simulink model "model"  (R2019a)
settings: Solver=ode15s  StartTime=0.0  StopTime=200  FixedStep=h  MaxStep=0.01  RelTol=1e-3
values from neighbouring files (symbols this model uses):
  d_cart = 4.3726    [parameters.m]
  d_pend = 0.0097    [parameters.m]
  g = 9.81    [parameters.m]
  h = 0.01    [parameters.m]
  Km = 3.7228    [parameters.m]
  l = 0.6    [parameters.m]
  mc = 0.5477    [parameters.m]
  mp = 0.0760    (= 0.076)    [parameters.m]
  sys = ss(A,B,C,D)    [linmod.m]
  ub_mtr_threshold = 0    [parameters.m]
  x_init = [0,0,0,0]    [parameters.m]
undefined symbols (not defined in the file or in its folder): K
libraries: cstblocks x3, mpclib x1
settings Model: Creator=mdepo  LastModifiedBy=mdepo

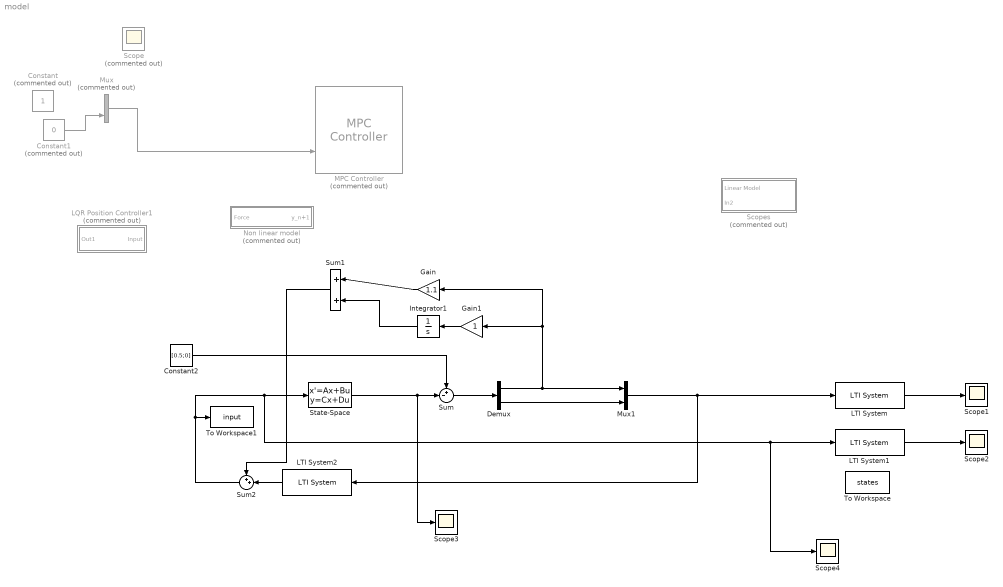
== system model ==
  Constant : Constant  Commented=on
  Constant1 : Constant  Commented=on  Value=0
  Constant2 : Constant  Value=[0.5;0]
  Demux : Demux  Outputs=2
  Gain : Gain  Gain=1.1
  Gain1 : Gain
  Integrator1 : Integrator
  LQR Position Controller1 : Subsystem  Commented=on
  LTI System : cstblocks/LTI System  sys=Ws  IC=[]
  LTI System1 : cstblocks/LTI System  sys=Wu  IC=[]
  LTI System2 : cstblocks/LTI System  sys=K  IC=[]
  MPC Controller : mpclib/MPC Controller  Commented=on  SCDEnableBlockLinearizationSpecification=on  mpcobj=mpcobj  is_multiple=0  enable_value=0  return_u0=off  updateMPCinCallerWorkspace=on  md_inport=off  mv_inport=off  uref_inport=off  return_cost=off  return_mvseq=off  return_qpstatus=off  return_xseq=off  return_state=off  return_ovseq=off  state_inport=off  umin_inport=off  umax_inport=off  ymin_inport=off  ymax_inport=off  cc_inport=off  ywt_inport=off  uwt_inport=off  duwt_inport=off  rhoeps_inport=off  pm_inport=off  MaximumP=10  HorizonChoice=FixedHorizon  n_ts=0.01  n_p=50  n_mv=1  n_md=0  n_ud=0  n_mo=1  n_uo=0  BlockDataType=double  SampleTimeInherited=off  switch_inport=off
      settings: SourceProductName=MATLAB Runtime - Model Predictive Control Toolbox Addin  SourceProductBaseCode=Missing
  Mux : Mux  Commented=on  Inputs=2
  Mux1 : Mux  Inputs=2
  Non linear model : Subsystem  Commented=on
  Scope : Scope  Commented=on
  Scope{1..4} (4 alike) : Scope
  "Scopes " : Subsystem  Commented=on
  State-Space : StateSpace  A=sys.A  B=sys.B  C=sys.C  D=sys.D  InitialCondition=x_init
  Sum : Sum  Inputs=+-|
  Sum1 : Sum  Inputs=|++
  Sum2 : Sum  Inputs=++|
  To Workspace : ToWorkspace  VariableName=states  SampleTime=h
  To Workspace1 : ToWorkspace  VariableName=input  SaveFormat=Timeseries  SampleTime=-1
  wires:
  Constant1/1 -> Mux/2
  Mux/1 -> MPC Controller/2
  LTI System/1 -> Scope1/1
  Constant2/1 -> Sum/1
  State-Space/1 -> Scope3/1, Sum/2
  LTI System1/1 -> Scope2/1
  Sum2/1 -> State-Space/1, Scope4/1, LTI System1/1, To Workspace1/1
  Sum/1 -> Demux/1
  Demux/2 -> Mux1/2
  Mux1/1 -> LTI System2/1, LTI System/1
  Demux/1 -> Gain/1, Gain1/1, Mux1/1
  Gain1/1 -> Integrator1/1
  LTI System2/1 -> Sum2/2
  Sum1/1 -> Sum2/1
  Integrator1/1 -> Sum1/2
  Gain/1 -> Sum1/1

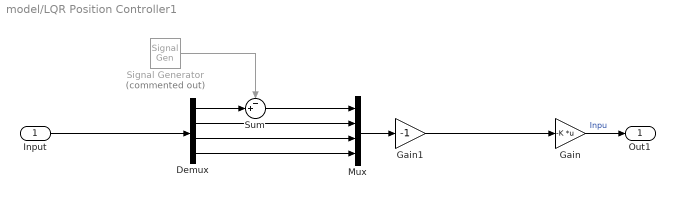
== system model/LQR Position Controller1 ==
  Input : Inport
  Demux : Demux
  Gain : Gain  Gain=-K  Multiplication=Matrix(K*u)
  Gain1 : Gain  Gain=-1
  Mux : Mux
  Signal Generator : SignalGenerator  Commented=on  Units=rad/sec
  Sum : Sum  Inputs=-+|
  Out1 : Outport
  wires:
  Signal Generator/1 -> Sum/1
  Sum/1 -> Mux/1
  Demux/1 -> Sum/2
  Mux/1 -> Gain1/1
  Input/1 -> Demux/1
  Demux/4 -> Mux/4
  Demux/3 -> Mux/3
  Demux/2 -> Mux/2
  Gain/1 -> Out1/1  "Inpu"
  Gain1/1 -> Gain/1

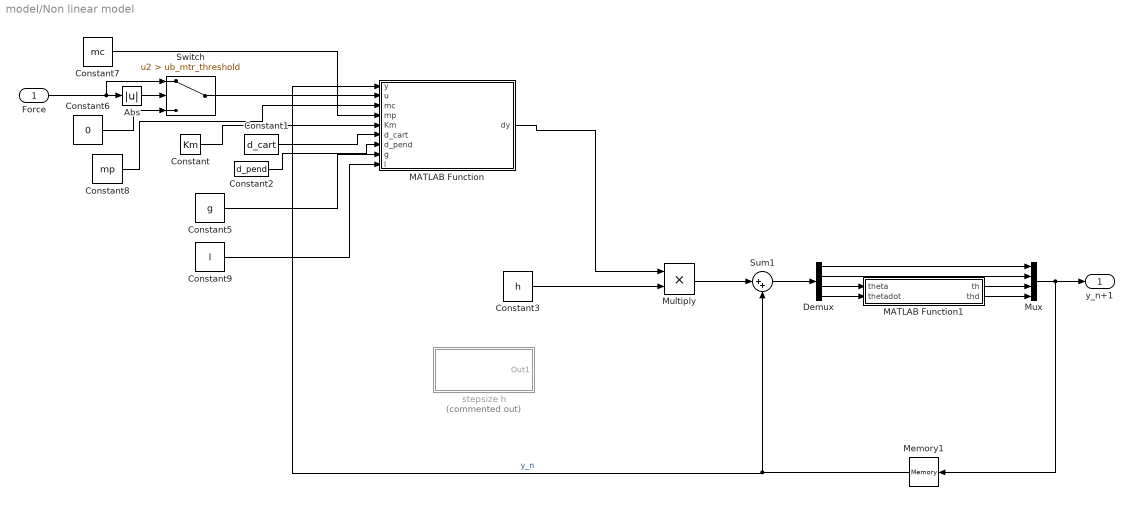
== system model/Non linear model ==
  Force : Inport
  Abs : Abs
  Constant : Constant  Value=Km
  Constant1 : Constant  Value=d_cart
  Constant2 : Constant  Value=d_pend
  Constant3 : Constant  Value=h  SampleTime=h
  Constant5 : Constant  Value=g
  Constant6 : Constant  Value=0
  Constant7 : Constant  Value=mc
  Constant8 : Constant  Value=mp
  Constant9 : Constant  Value=l
  Demux : Demux
  MATLAB Function : MATLAB Function  TreatAsAtomicUnit=on
  MATLAB Function1 : MATLAB Function  TreatAsAtomicUnit=on
  Memory1 : Memory  InitialCondition=x_init
  Multiply : Product
  Mux : Mux
  Sum1 : Sum  Inputs=|++
  Switch : Switch  Criteria=u2 > Threshold  Threshold=ub_mtr_threshold
  stepsize h : Subsystem  Commented=on
  y_n+1 : Outport
  wires:
  Abs/1 -> Switch/2
  Constant5/1 -> MATLAB Function/8(g)
  Constant6/1 -> Switch/3
  Sum1/1 -> Demux/1
  Mux/1 -> Memory1/1, y_n+1/1
  Constant3/1 -> Multiply/2
  Constant2/1 -> MATLAB Function/7(d_pend)
  Constant/1 -> MATLAB Function/5(Km)
  Memory1/1 -> MATLAB Function/1(y), Sum1/2  "y_n"
  MATLAB Function/1(dy) -> Multiply/1
  Demux/2 -> Mux/2
  Constant1/1 -> MATLAB Function/6(d_cart)
  Demux/1 -> Mux/1
  Force/1 -> Abs/1, Switch/1
  Multiply/1 -> Sum1/1
  Switch/1 -> MATLAB Function/2(u)
  Constant8/1 -> MATLAB Function/3(mc)
  Constant7/1 -> MATLAB Function/4(mp)
  Constant9/1 -> MATLAB Function/9(l)
  Demux/4 -> MATLAB Function1/2(thetadot)
  Demux/3 -> MATLAB Function1/1(theta)
  MATLAB Function1/1(th) -> Mux/3
  MATLAB Function1/2(thd) -> Mux/4

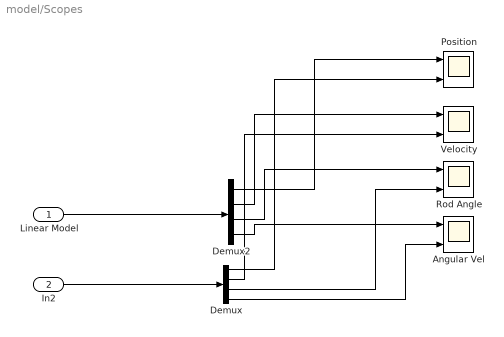
== system model/Scopes  ==
  Linear Model : Inport
  In2 : Inport  Port=2
  "Angular Vel " : Scope  NumInputPorts=2
  Demux : Demux
  Demux2 : Demux
  Position : Scope  NumInputPorts=2
  Rod Angle : Scope  NumInputPorts=2
  Velocity : Scope  NumInputPorts=2
  wires:
  Linear Model/1 -> Demux2/1
  Demux2/1 -> Position/1
  Demux2/2 -> Velocity/1
  Demux2/3 -> Rod Angle/1
  Demux2/4 -> "Angular Vel "/1
  In2/1 -> Demux/1
  Demux/1 -> Position/2
  Demux/2 -> Velocity/2
  Demux/3 -> Rod Angle/2
  Demux/4 -> "Angular Vel "/2

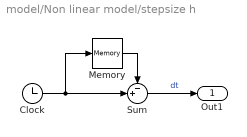
== system model/Non linear model/stepsize h ==
  Clock : Clock
  Memory : Memory
  Sum : Sum  Inputs=-+|
  Out1 : Outport
  wires:
  Memory/1 -> Sum/1
  Sum/1 -> Out1/1  "dt"
  Clock/1 -> Memory/1, Sum/2

== matlab function model/Non linear model/MATLAB Function1 ==
  data: theta input; th output; thetadot input; thd output
function [th,thd] = fcn(theta, thetadot)

threshold = 0.26;

if abs(theta) > threshold
    th = threshold;
    thd = 0;
else
    th = theta;
    thd = thetadot;
end

== matlab function model/Non linear model/MATLAB Function ==
  data: y input; u input; dy output; mc input; mp input; Km input; d_cart input; d_pend input; g input; l input
function dy = fcn(y,u,mc,mp,Km,d_cart,d_pend,g,l)
dy = zeros(4,1);
dy(1,1) = y(2);
dy(2,1) = 1/((mc+mp)*(1-0.75*mp))*(Km*u - d_cart*y(2) + 3/(2*l)*((l/2)*mp*g*y(3) - d_pend*y(4)) + 0*mp*l*y(4)^2*y(3)/2);
dy(3,1) = y(4);
dy(4,1) = 3/(mp*l^2)*(l*mp*dy(2,1)/2 + l*mp*g*y(3)/2 - d_pend*y(4));
end
